simulink model "SNS_SpikingRG_MN"  (R2025a)
settings: Solver=ode45  StartTime=0.0  StopTime=12  RelTol=1e-3
libraries: SNS_Library x23
settings Model: Creator=Ben Bolen  LastModifiedBy=Ben Bolen

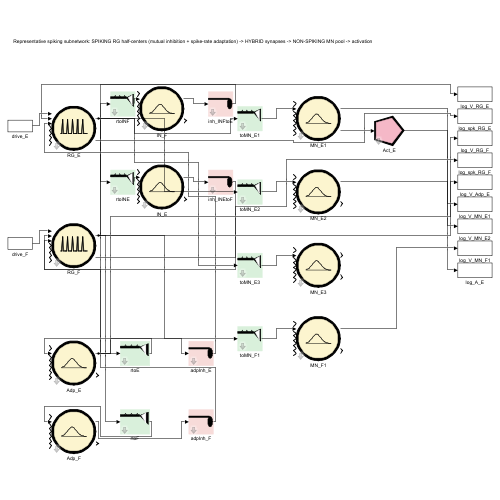
[thumbnail: Simulink's stored preview of the top-level diagram]
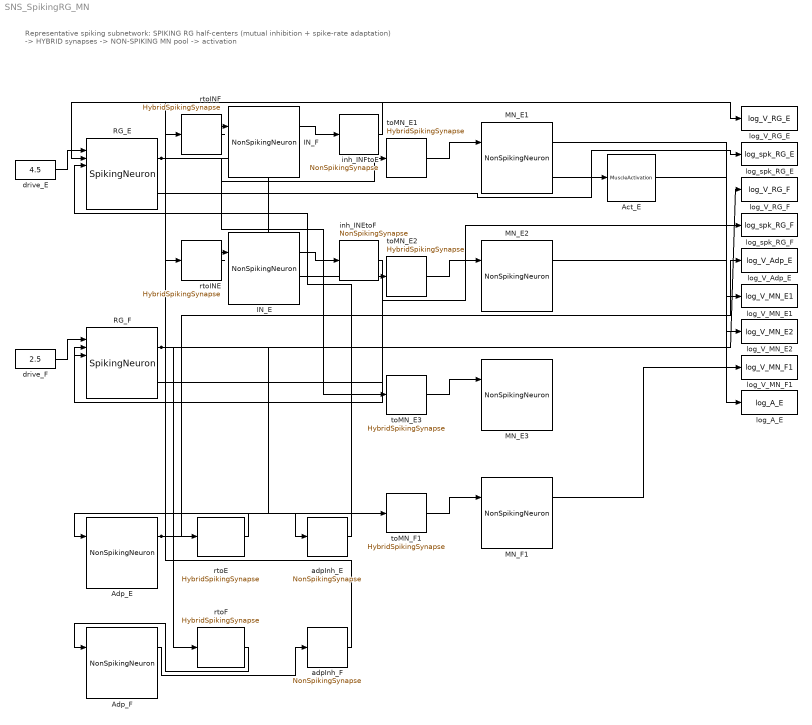
== system SNS_SpikingRG_MN ==
  note: Representative spiking subnetwork: SPIKING RG half-centers (mutual inhibition + spike-rate adaptation) -> HYBRID synapses -> NON-SPIKING MN pool -> activation
  Act_E : SNS_Library/MuscleActivation  tauAct=50  A0=0
  Adp_E : SNS_Library/NonSpikingNeuron  Vrest=-52  Gm=0.1  Cm=40  Thr=-55  Slope=1
  Adp_F : SNS_Library/NonSpikingNeuron  Vrest=-52  Gm=0.1  Cm=40  Thr=-55  Slope=1
  IN_E : SNS_Library/NonSpikingNeuron  Vrest=-52  Gm=0.1  Cm=5  Thr=-55  Slope=1
  IN_F : SNS_Library/NonSpikingNeuron  Vrest=-52  Gm=0.1  Cm=5  Thr=-55  Slope=1
  MN_E1 : SNS_Library/NonSpikingNeuron  Vrest=-52  Gm=0.5  Cm=5  Thr=-45  Slope=1
  MN_E2 : SNS_Library/NonSpikingNeuron  Vrest=-52  Gm=0.5  Cm=5  Thr=-45  Slope=1
  MN_E3 : SNS_Library/NonSpikingNeuron  Vrest=-52  Gm=0.5  Cm=5  Thr=-45  Slope=1
  MN_F1 : SNS_Library/NonSpikingNeuron  Vrest=-52  Gm=0.5  Cm=5  Thr=-45  Slope=1
  RG_E : SNS_Library/SpikingNeuron  Vrest=-52  Vth=-45  Vreset=-60  Gm=0.1  Cm=5
  RG_F : SNS_Library/SpikingNeuron  Vrest=-52  Vth=-45  Vreset=-60  Gm=0.1  Cm=5
  adpInh_E : SNS_Library/NonSpikingSynapse  gmax=0.3  Esyn=-80  ThrPre=-45  SlopePre=0.5
  adpInh_F : SNS_Library/NonSpikingSynapse  gmax=0.3  Esyn=-80  ThrPre=-45  SlopePre=0.5
  drive_E : Constant  Value=4.5
  drive_F : Constant  Value=2.5
  inh_INEtoF : SNS_Library/NonSpikingSynapse  gmax=0.2  Esyn=-80  ThrPre=-45  SlopePre=0.5
  inh_INFtoE : SNS_Library/NonSpikingSynapse  gmax=0.2  Esyn=-80  ThrPre=-45  SlopePre=0.5
  log_A_E : ToWorkspace  VariableName=log_A_E  SaveFormat=Timeseries  SampleTime=-1
  log_V_Adp_E : ToWorkspace  VariableName=log_V_Adp_E  SaveFormat=Timeseries  SampleTime=-1
  log_V_MN_E1 : ToWorkspace  VariableName=log_V_MN_E1  SaveFormat=Timeseries  SampleTime=-1
  log_V_MN_E2 : ToWorkspace  VariableName=log_V_MN_E2  SaveFormat=Timeseries  SampleTime=-1
  log_V_MN_F1 : ToWorkspace  VariableName=log_V_MN_F1  SaveFormat=Timeseries  SampleTime=-1
  log_V_RG_E : ToWorkspace  VariableName=log_V_RG_E  SaveFormat=Timeseries  SampleTime=-1
  log_V_RG_F : ToWorkspace  VariableName=log_V_RG_F  SaveFormat=Timeseries  SampleTime=-1
  log_spk_RG_E : ToWorkspace  VariableName=log_spk_RG_E  SaveFormat=Timeseries  SampleTime=-1
  log_spk_RG_F : ToWorkspace  VariableName=log_spk_RG_F  SaveFormat=Timeseries  SampleTime=-1
  rtoE : SNS_Library/HybridSpikingSynapse  gmax=1.0  ginc=0.05  tau_syn=150  Esyn=0  ThrPre=-47
  rtoF : SNS_Library/HybridSpikingSynapse  gmax=1.0  ginc=0.05  tau_syn=150  Esyn=0  ThrPre=-47
  rtoINE : SNS_Library/HybridSpikingSynapse  gmax=0.5  ginc=0.1  tau_syn=100  Esyn=0  ThrPre=-47
  rtoINF : SNS_Library/HybridSpikingSynapse  gmax=0.5  ginc=0.1  tau_syn=100  Esyn=0  ThrPre=-47
  toMN_E1 : SNS_Library/HybridSpikingSynapse  gmax=0.5  ginc=0.05  tau_syn=20  Esyn=0  ThrPre=-47
  toMN_E2 : SNS_Library/HybridSpikingSynapse  gmax=0.5  ginc=0.05  tau_syn=20  Esyn=0  ThrPre=-47
  toMN_E3 : SNS_Library/HybridSpikingSynapse  gmax=0.5  ginc=0.05  tau_syn=20  Esyn=0  ThrPre=-47
  toMN_F1 : SNS_Library/HybridSpikingSynapse  gmax=0.5  ginc=0.05  tau_syn=20  Esyn=0  ThrPre=-47
  wires:
  drive_E/1 -> RG_E/1
  drive_F/1 -> RG_F/1
  RG_E/1 -> rtoINE/1, rtoE/1, toMN_E1/1, toMN_E2/1, toMN_E3/1, log_V_RG_E/1
  RG_F/1 -> rtoINF/1, rtoF/1, toMN_F1/1, log_V_RG_F/1
  rtoINE/1 -> IN_E/2
  rtoINF/1 -> IN_F/2
  IN_E/1 -> inh_INEtoF/1
  IN_F/1 -> inh_INFtoE/1
  inh_INEtoF/1 -> RG_F/2
  inh_INFtoE/1 -> RG_E/2
  rtoE/1 -> Adp_E/2
  rtoF/1 -> Adp_F/2
  Adp_E/1 -> adpInh_E/1, log_V_Adp_E/1
  Adp_F/1 -> adpInh_F/1
  adpInh_E/1 -> RG_E/3
  adpInh_F/1 -> RG_F/3
  toMN_E1/1 -> MN_E1/2
  toMN_E2/1 -> MN_E2/2
  toMN_E3/1 -> MN_E3/2
  toMN_F1/1 -> MN_F1/2
  MN_E1/2 -> Act_E/1
  RG_E/2 -> log_spk_RG_E/1
  RG_F/2 -> log_spk_RG_F/1
  MN_E1/1 -> log_V_MN_E1/1
  MN_E2/1 -> log_V_MN_E2/1
  MN_F1/1 -> log_V_MN_F1/1
  Act_E/1 -> log_A_E/1
